simulink model "VS_AWD_Status_Model"  (R2024a)
settings: Solver=FixedStepDiscrete  StartTime=0.0  StopTime=10.0  FixedStep=0.01  RelTol=1e-3  EnableMultiTasking=on
undefined symbols (not defined in the file or in its folder): kZero_s16
settings Model: DataDictionary=VS_AWD_Status_DD.sldd  Creator=shanba  LastModifiedBy=sasi.kakarla_methodi
settings ConfigSet: Description="This Simulink Configuration Set is preconfigured  for the MotoHawk target \"ECM-5554-112-0904-xD\"."
settings SolverCC: AlgebraicLoopSolver=TrustRegion
settings DataIOCC: LimitDataPoints=on  SaveFormat=Array  ReturnWorkspaceOutputs=off
settings OptimizationCC: DefaultUnderspecifiedDataType=single  EnhancedBackFolding=on  PassReuseOutputArgsAs=Individual arguments  InitFltsAndDblsToZero=on  EfficientFloat2IntCast=on  OptimizeBlockOrder=speed  DifferentSizesBufferReuse=on  OptimizationCustomize=off  EfficientTunableParamExpr=on
settings DebuggingCC: MergeDetectMultiDrivingBlocksExec=none  InheritedTsInSrcMsg=none  MultiTaskDSMMsg=none  TasksWithSamePriorityMsg=none  ParameterPrecisionLossMsg=none  ParameterTunabilityLossMsg=error  UnconnectedInputMsg=warning  UnconnectedOutputMsg=warning  UnconnectedLineMsg=warning  ModelReferenceIOMismatchMessage=warning  SFExecutionAtInitializationDiag=none  ArithmeticOperatorsInVariantConditions=warning
settings HardwareCC: ProdBitPerPointer=32  ProdBitPerSizeT=32  ProdBitPerPtrDiffT=32  ProdLargestAtomicFloat=None  ProdWordSize=32  ProdHWDeviceType=Infineon->TriCore
settings ModelReferenceCC: UpdateModelReferenceTargets=IfOutOfDate  EnableRefExpFcnMdlSchedulingChecks=on  CheckModelReferenceTargetMessage=warning  ModelReferenceNumInstancesAllowed=Single  PropagateSignalLabelsOutOfModel=off
settings SFSimCC: SimUseLocalCustomCode=off  SimGenImportedTypeDefs=on  CompileTimeRecursionLimit=100  LegacyBehaviorForPersistentVarInContinuousTime=on  CustomCodeUndefinedFunction=UseInterfaceOnly  CustomCodeGlobalsAsFunctionIO=on  DefaultCustomCodeDeterministicFunctions=All
settings RTWCC: Description=Embedded Coder  SystemTargetFile=ert.tlc  EmbeddedCoderDictionary=EmbeddedCoderDictionary.sldd  GenCodeOnly=on  TemplateMakefile=ert_default_tmf  GenerateReport=on  RTWUseLocalCustomCode=off  IncludeHyperlinkInReport=on  LaunchReport=on  GenerateTraceInfo=on  GenerateTraceReport=on  GenerateCodeMetricsReport=on  GenerateCodeReplacementReport=on  GPUComputeCapability=3.5
settings CodeAppCC: ForceParamTrailComments=on  IgnoreCustomStorageClasses=off  MaxIdLength=100  OperatorAnnotations=on  SimulinkDataObjDesc=on  SFDataObjDesc=on  CustomSymbolStrTmpVar=$R$N$M  InsertBlockDesc=on
settings ERTTargetCC: TargetLangStandard=C99 (ISO)  GenerateSampleERTMain=on  SupportNonFinite=off  ERTSrcFileBannerTemplate=ert_code_fsw.cgt  ERTHdrFileBannerTemplate=ert_code_fsw.cgt  ERTDataSrcFileTemplate=ert_code_fsw.cgt  ERTDataHdrFileTemplate=ert_code_fsw.cgt  ERTCustomFileTemplate=example_file_process.tlc  EnableUserReplacementTypes=on
settings ConfigComp: CovMetricSettings=dw  CovSaveCumulativeToWorkspaceVar=on  CovSaveSingleToWorkspaceVar=on  CovExternalEMLEnable=off  CovSFcnEnable=off

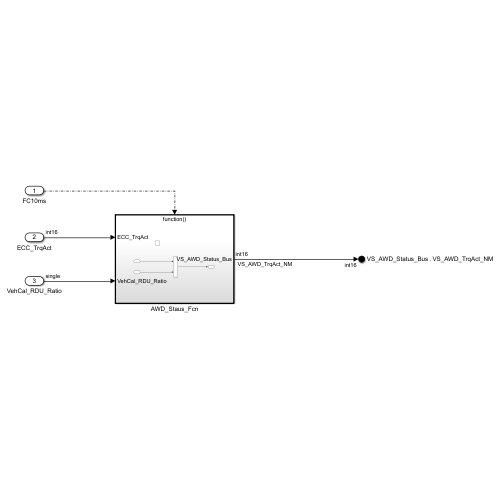
[thumbnail: Simulink's stored preview of the top-level diagram]
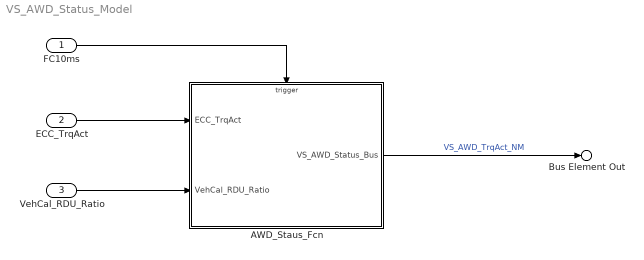
== system VS_AWD_Status_Model ==
  FC10ms : Inport  OutDataTypeStr=single  PortDimensions=1  OutputFunctionCall=on
  ECC_TrqAct : Inport  Port=2  OutDataTypeStr=int16  PortDimensions=1
  VehCal_RDU_Ratio : Inport  Port=3  OutDataTypeStr=single  PortDimensions=1
  AWD_Staus_Fcn : Subsystem  TreatAsAtomicUnit=on
  Bus Element Out : Outport  PortName=VS_AWD_Status_Bus  Element=VS_AWD_TrqAct_NM
  wires:
  AWD_Staus_Fcn/1(VS_AWD_Status_Bus) -> Bus Element Out/1  "VS_AWD_TrqAct_NM"
  ECC_TrqAct/1 -> AWD_Staus_Fcn/1(ECC_TrqAct)
  VehCal_RDU_Ratio/1 -> AWD_Staus_Fcn/2(VehCal_RDU_Ratio)
  FC10ms/1 -> AWD_Staus_Fcn/Trigger

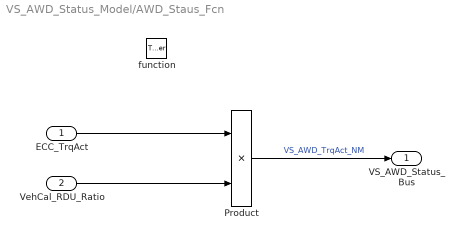
== system VS_AWD_Status_Model/AWD_Staus_Fcn ==
  ECC_TrqAct : Inport
  VehCal_RDU_Ratio : Inport  Port=2
  function : TriggerPort  TriggerType=function-call  VariantControl=(inherit)
  Product : Product  OutDataTypeStr=Inherit: Same as first input
  VS_AWD_Status_Bus : Outport  InitialOutput=kZero_s16
  wires:
  Product/1 -> VS_AWD_Status_Bus/1  "VS_AWD_TrqAct_NM"
  VehCal_RDU_Ratio/1 -> Product/2
  ECC_TrqAct/1 -> Product/1
